simulink model "hinf_arduino"  (R2015a)
settings: Solver=ode3  StartTime=0.0  StopTime=10.0  FixedStep=1/200  RelTol=1e-3
values from neighbouring files (symbols this model uses):
  Hinf = ss(Hinf_red)    [controller_parameters.m]
libraries: PoliArd x9, simulink x6
settings Model: ExtModeTrigDuration=2  Creator=GSavaia  LastModifiedBy=user
settings OptimizationCC: OptimizeModelRefInitCode=on  LifeSpan=1
settings DebuggingCC: UnderspecifiedInitializationDetection=Classic  MergeDetectMultiDrivingBlocksExec=none
settings HardwareCC: ProdLargestAtomicInteger=Long  ProdLargestAtomicFloat=Double  ProdEndianess=LittleEndian  ProdHWDeviceType=ARM Compatible->ARM Cortex
settings RTWCC: SystemTargetFile=realtime.tlc  GenerateMakefile=off  TemplateMakefile=realtime.tmf  Description=Run on Target Hardware  RTWVerbose=off
settings ERTTargetCC: CombineOutputUpdateFcns=off  ExtModeTransport=3  ExtModeMexFile=ext_serial_win32_comm_rtt  ExtModeMexArgs=0 1 9600  ERTSrcFileBannerTemplate=realtime_code_template.cgt  ERTHdrFileBannerTemplate=realtime_code_template.cgt  ERTDataSrcFileTemplate=realtime_code_template.cgt  ERTDataHdrFileTemplate=realtime_code_template.cgt  ERTCustomFileTemplate=realtime_file_process.tlc

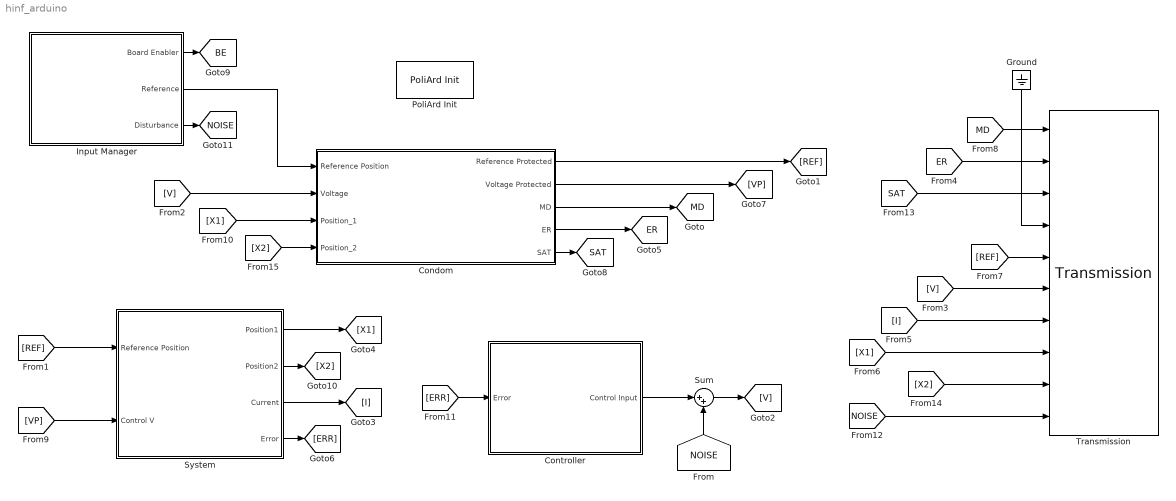
== system hinf_arduino ==
  Condom : Subsystem
  Controller : Subsystem
  Ground : Ground
  Input Manager : Subsystem
  PoliArd Init : PoliArd/PoliArd Init
  Sum : Sum  Inputs=|++
  "System " : Subsystem
  Transmission : PoliArd/Transmission  sample_freq=200  sig_to_send=6
  tag scope: BE=global, ER=global, MD=global, NOISE=global, SAT=global
  wires:
  Condom/1(Reference Protected) -> [REF]
  [REF] -> "System "/1(Reference Position)
  "System "/3(Current) -> [I]
  [V] -> Condom/2(Voltage)
  [V] -> Transmission/6
  [I] -> Transmission/7
  "System "/1(Position1) -> [X1]
  [REF] -> Transmission/5
  [MD] -> Transmission/1
  [VP] -> "System "/2(Control V)
  [X1] -> Condom/3(Position_1)
  [X1] -> Transmission/8
  "System "/4(Error) -> [ERR]
  [ERR] -> Controller/1(Error)
  Condom/2("Voltage Protected ") -> [VP]
  Condom/3(MD) -> [MD]
  Condom/4(ER) -> [ER]
  Ground/1 -> Transmission/4
  [ER] -> Transmission/2
  [SAT] -> Transmission/3
  Condom/5(SAT) -> [SAT]
  Sum/1 -> [V]
  Controller/1(Control Input) -> Sum/1
  [NOISE] -> Sum/2
  Input Manager/1(Board Enabler) -> [BE]
  Input Manager/3(Disturbance) -> [NOISE]
  Input Manager/2(Reference) -> Condom/1(Reference Position)
  "System "/2(Position2) -> [X2]
  [NOISE] -> Transmission/10
  [X2] -> Condom/4(Position_2)
  [X2] -> Transmission/9

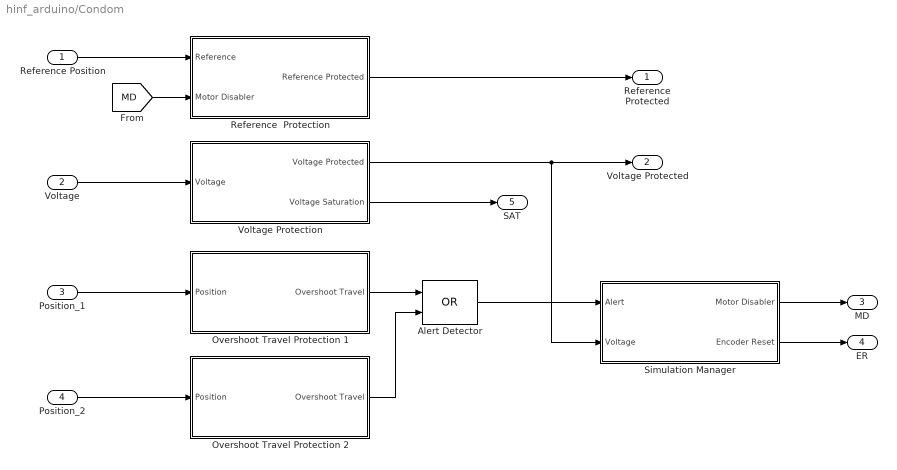
== system hinf_arduino/Condom ==
  Reference Position : Inport
  Voltage : Inport  Port=2
  Position_1 : Inport  Port=3
  Position_2 : Inport  Port=4
  Alert Detector : Logic  Operator=OR  AllPortsSameDT=off  OutDataTypeStr=boolean
  Overshoot Travel Protection 1 : Subsystem
  Overshoot Travel Protection 2 : Subsystem
  Reference  Protection : Subsystem
  Simulation Manager : Subsystem
  Voltage Protection : Subsystem
  Reference Protected : Outport
  "Voltage Protected " : Outport  Port=2
  MD : Outport  Port=3
  ER : Outport  Port=4
  SAT : Outport  Port=5
  wires:
  Reference Position/1 -> Reference  Protection/1("Reference ")
  Position_1/1 -> Overshoot Travel Protection 1/1("Position ")
  Overshoot Travel Protection 1/1(Overshoot Travel) -> Alert Detector/1
  Voltage/1 -> Voltage Protection/1("Voltage ")
  Voltage Protection/1(Voltage Protected) -> Simulation Manager/2(Voltage), "Voltage Protected "/1
  Reference  Protection/1(Reference Protected) -> Reference Protected/1
  Alert Detector/1 -> Simulation Manager/1(Alert)
  Simulation Manager/2(Encoder Reset) -> ER/1
  Simulation Manager/1(Motor Disabler) -> MD/1
  [MD] -> Reference  Protection/2(Motor Disabler)
  Voltage Protection/2(Voltage Saturation) -> SAT/1
  Position_2/1 -> Overshoot Travel Protection 2/1("Position ")
  Overshoot Travel Protection 2/1(Overshoot Travel) -> Alert Detector/2

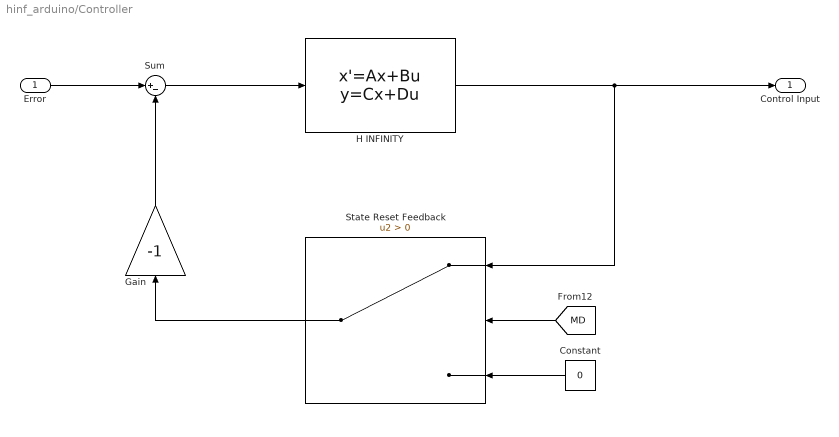
== system hinf_arduino/Controller ==
  Error : Inport
  Constant : Constant  Value=0
  Gain : Gain  Gain=-1
  H INFINITY : StateSpace  A=Hinf.A  B=Hinf.B  C=Hinf.C  D=Hinf.D  X0=0
  State Reset Feedback : Switch  Criteria=u2 > Threshold
  Sum : Sum  Inputs=|+-
  Control Input : Outport
  wires:
  H INFINITY/1 -> State Reset Feedback/1, Control Input/1
  Error/1 -> Sum/1
  Sum/1 -> H INFINITY/1
  Constant/1 -> State Reset Feedback/3
  Gain/1 -> Sum/2
  State Reset Feedback/1 -> Gain/1
  [MD] -> State Reset Feedback/2

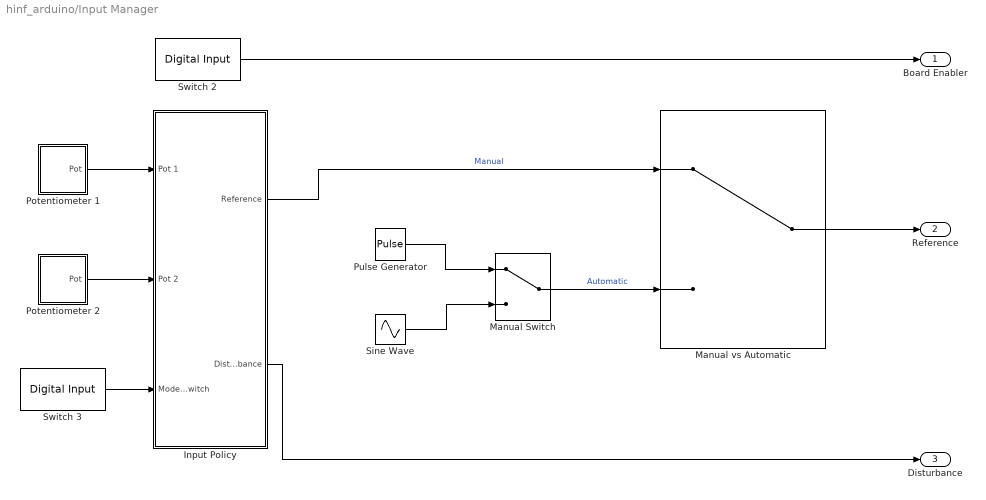
== system hinf_arduino/Input Manager ==
  Input Policy : Subsystem
  Manual vs Automatic : ManualSwitch
  Manual Switch : ManualSwitch
  Potentiometer 1 : Subsystem
  Potentiometer 2 : Subsystem
  Pulse Generator : DiscretePulseGenerator  PulseType=Time based  Amplitude=2  Period=10  PulseWidth=50
  Sine Wave : Sin  Amplitude=0.5  Bias=0.7  Frequency=pi  SampleTime=0
  Switch 2 : PoliArd/Digital Input  DI_pin=2  DIsample=-1
  Switch 3 : PoliArd/Digital Input  DI_pin=3  DIsample=-1
  Board Enabler : Outport
  Reference : Outport  Port=2
  Disturbance : Outport  Port=3
  wires:
  Switch 2/1 -> Board Enabler/1
  Switch 3/1 -> Input Policy/3(Mode Switch)
  Pulse Generator/1 -> Manual Switch/1
  Sine Wave/1 -> Manual Switch/2
  Potentiometer 1/1(Pot) -> Input Policy/1(Pot 1)
  Potentiometer 2/1(Pot) -> Input Policy/2(Pot 2)
  Input Policy/1(Reference) -> Manual vs Automatic/1  "Manual"
  Manual Switch/1 -> Manual vs Automatic/2  "Automatic"
  Input Policy/2(Disturbance) -> Disturbance/1
  Manual vs Automatic/1 -> Reference/1

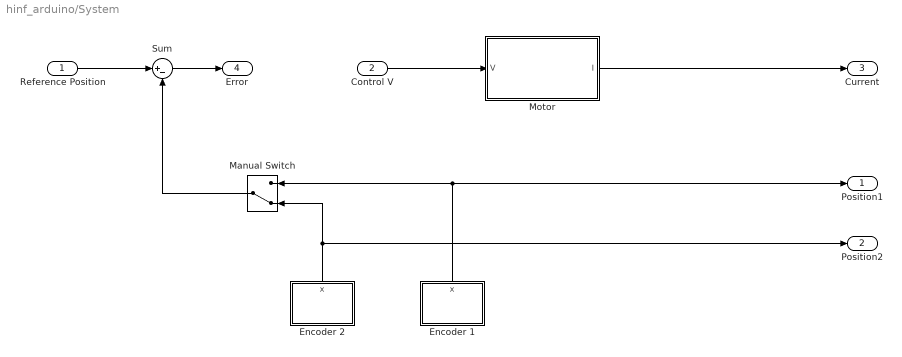
== system hinf_arduino/System  ==
  Reference Position : Inport
  Control V : Inport  Port=2
  "Encoder 1 " : Subsystem
  Encoder 2 : Subsystem
  Manual Switch : ManualSwitch  CurrentSetting=0
  Motor : Subsystem
  Sum : Sum  Inputs=|+-
  Position1 : Outport
  Position2 : Outport  Port=2
  Current : Outport  Port=3
  Error : Outport  Port=4
  wires:
  Reference Position/1 -> Sum/1
  Motor/1(I) -> Current/1
  Sum/1 -> Error/1
  Control V/1 -> Motor/1(V)
  Manual Switch/1 -> Sum/2
  Encoder 2/1(x) -> Position2/1, Manual Switch/2
  "Encoder 1 "/1(x) -> Manual Switch/1, Position1/1

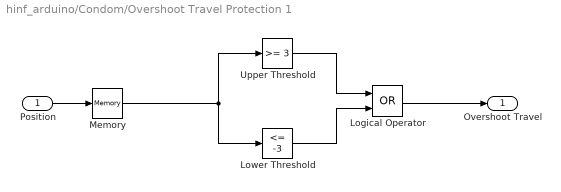
== system hinf_arduino/Condom/Overshoot Travel Protection 1 ==
  "Position " : Inport
  Logical Operator : Logic  Operator=OR  AllPortsSameDT=off  OutDataTypeStr=boolean
  Lower Threshold : simulink/Logic and Bit Operations/Compare To Constant  relop=<=  const=-3  OutDataTypeStr=boolean
  Memory : Memory  InheritSampleTime=on
  Upper Threshold : simulink/Logic and Bit Operations/Compare To Constant  relop=>=  const=3  OutDataTypeStr=boolean
  Overshoot Travel : Outport
  wires:
  Logical Operator/1 -> Overshoot Travel/1
  Lower Threshold/1 -> Logical Operator/2
  Upper Threshold/1 -> Logical Operator/1
  "Position "/1 -> Memory/1
  Memory/1 -> Lower Threshold/1, Upper Threshold/1

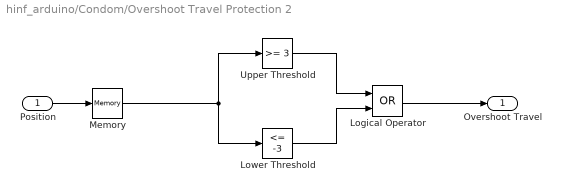
== system hinf_arduino/Condom/Overshoot Travel Protection 2 ==
  "Position " : Inport
  Logical Operator : Logic  Operator=OR  AllPortsSameDT=off  OutDataTypeStr=boolean
  Lower Threshold : simulink/Logic and Bit Operations/Compare To Constant  relop=<=  const=-3  OutDataTypeStr=boolean
  Memory : Memory  InheritSampleTime=on
  Upper Threshold : simulink/Logic and Bit Operations/Compare To Constant  relop=>=  const=3  OutDataTypeStr=boolean
  Overshoot Travel : Outport
  wires:
  Logical Operator/1 -> Overshoot Travel/1
  Lower Threshold/1 -> Logical Operator/2
  Upper Threshold/1 -> Logical Operator/1
  "Position "/1 -> Memory/1
  Memory/1 -> Lower Threshold/1, Upper Threshold/1

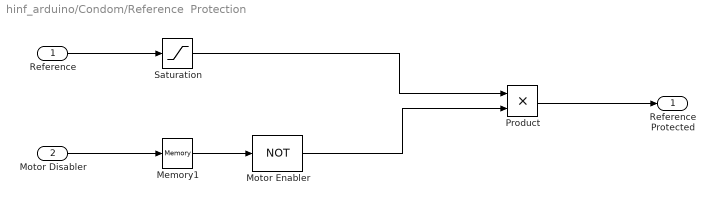
== system hinf_arduino/Condom/Reference  Protection ==
  "Reference " : Inport
  Motor Disabler : Inport  Port=2
  Memory1 : Memory  X0=1  InheritSampleTime=on
  Motor Enabler : Logic  Operator=NOT  Inputs=1  AllPortsSameDT=off  OutDataTypeStr='double'
  Product : Product
  Saturation : Saturate  UpperLimit=3  LowerLimit=-3
  Reference Protected : Outport
  wires:
  "Reference "/1 -> Saturation/1
  Saturation/1 -> Product/1
  Motor Enabler/1 -> Product/2
  Memory1/1 -> Motor Enabler/1
  Product/1 -> Reference Protected/1
  Motor Disabler/1 -> Memory1/1

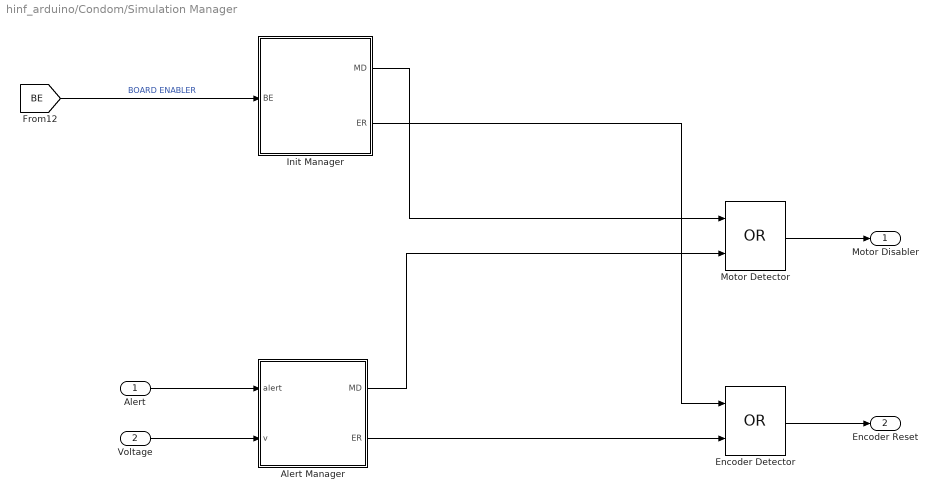
== system hinf_arduino/Condom/Simulation Manager ==
  Alert : Inport
  Voltage : Inport  Port=2
  Alert Manager : Stateflow chart  TreatAsAtomicUnit=on
  Encoder Detector : Logic  Operator=OR  AllPortsSameDT=off  OutDataTypeStr=boolean
  Init Manager : Stateflow chart  TreatAsAtomicUnit=on
  Motor Detector : Logic  Operator=OR  AllPortsSameDT=off  OutDataTypeStr=boolean
  Motor Disabler : Outport
  Encoder Reset : Outport  Port=2
  wires:
  [BE] -> Init Manager/1(BE)  "BOARD ENABLER"
  Motor Detector/1 -> Motor Disabler/1
  Encoder Detector/1 -> Encoder Reset/1
  Init Manager/1(MD) -> Motor Detector/1
  Alert Manager/1(MD) -> Motor Detector/2
  Init Manager/2(ER) -> Encoder Detector/1
  Alert Manager/2(ER) -> Encoder Detector/2
  Alert/1 -> Alert Manager/1(alert)
  Voltage/1 -> Alert Manager/2(v)

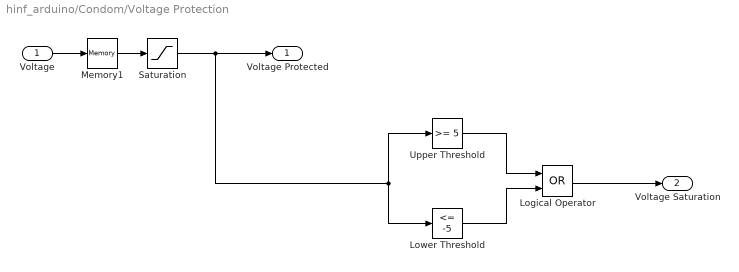
== system hinf_arduino/Condom/Voltage Protection ==
  "Voltage " : Inport
  Logical Operator : Logic  Operator=OR  AllPortsSameDT=off  OutDataTypeStr=boolean
  Lower Threshold : simulink/Logic and Bit Operations/Compare To Constant  relop=<=  const=-5  OutDataTypeStr=boolean
  Memory1 : Memory  InheritSampleTime=on
  Saturation : Saturate  UpperLimit=5  LowerLimit=-5
  Upper Threshold : simulink/Logic and Bit Operations/Compare To Constant  relop=>=  const=5  OutDataTypeStr=boolean
  Voltage Protected : Outport
  Voltage Saturation : Outport  Port=2
  wires:
  "Voltage "/1 -> Memory1/1
  Logical Operator/1 -> Voltage Saturation/1
  Lower Threshold/1 -> Logical Operator/2
  Upper Threshold/1 -> Logical Operator/1
  Saturation/1 -> Lower Threshold/1, Upper Threshold/1, Voltage Protected/1
  Memory1/1 -> Saturation/1

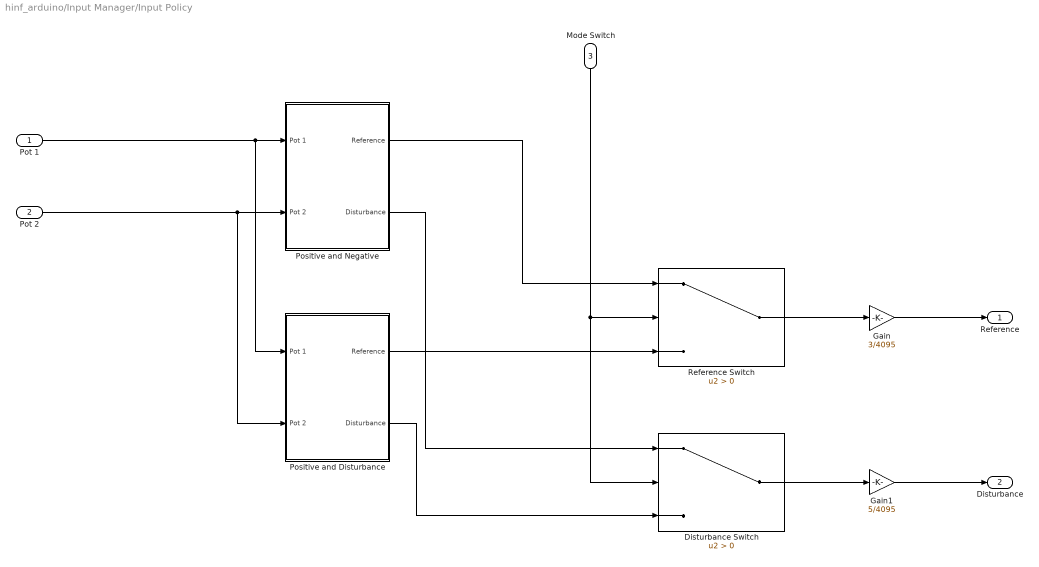
== system hinf_arduino/Input Manager/Input Policy ==
  Pot 1 : Inport
  Pot 2 : Inport  Port=2
  Mode Switch : Inport  Port=3
  Disturbance Switch : Switch  Criteria=u2 > Threshold
  Gain : Gain  Gain=3/4095
  Gain1 : Gain  Gain=5/4095
  Positive and Disturbance : Subsystem
  Positive and Negative : Subsystem
  Reference Switch : Switch  Criteria=u2 > Threshold
  Reference : Outport
  Disturbance : Outport  Port=2
  wires:
  Pot 1/1 -> Positive and Disturbance/1(Pot 1), Positive and Negative/1(Pot 1)
  Pot 2/1 -> Positive and Disturbance/2(Pot 2), Positive and Negative/2(Pot 2)
  Mode Switch/1 -> Reference Switch/2, Disturbance Switch/2
  Reference Switch/1 -> Gain/1
  Disturbance Switch/1 -> Gain1/1
  Positive and Negative/1(Reference) -> Reference Switch/1
  Positive and Disturbance/1(Reference) -> Reference Switch/3
  Positive and Negative/2(Disturbance) -> Disturbance Switch/1
  Positive and Disturbance/2(Disturbance) -> Disturbance Switch/3
  Gain/1 -> Reference/1
  Gain1/1 -> Disturbance/1

== system hinf_arduino/Input Manager/Potentiometer 1 ==
  Analog Input : PoliArd/Analog Input  AIpin_mask=8  AIsample=-1
  Data Type Conversion1 : DataTypeConversion
  Transfer Fcn : TransferFcn  Numerator=1  Denominator=[1/(2*pi*5) 1]
  Pot : Outport
  wires:
  Analog Input/1 -> Data Type Conversion1/1
  Transfer Fcn/1 -> Pot/1
  Data Type Conversion1/1 -> Transfer Fcn/1

== system hinf_arduino/Input Manager/Potentiometer 2 ==
  Analog Input : PoliArd/Analog Input  AIpin_mask=9  AIsample=-1
  Data Type Conversion1 : DataTypeConversion
  Transfer Fcn : TransferFcn  Numerator=1  Denominator=[1/(2*pi*5) 1]
  Pot : Outport
  wires:
  Analog Input/1 -> Data Type Conversion1/1
  Transfer Fcn/1 -> Pot/1
  Data Type Conversion1/1 -> Transfer Fcn/1

== system hinf_arduino/System /Encoder 1  ==
  Encoder : PoliArd/Encoder  EncoderID=1  dt_enc=1/200
  encoder-to-cm : Gain  Gain=1/560
  x : Outport
  wires:
  Encoder/1 -> encoder-to-cm/1
  [ER] -> Encoder/1
  encoder-to-cm/1 -> x/1

== system hinf_arduino/System /Encoder 2 ==
  Encoder : PoliArd/Encoder  EncoderID=4  dt_enc=1/200
  encoder-to-cm : Gain  Gain=1/560
  x : Outport
  wires:
  Encoder/1 -> encoder-to-cm/1
  [ER] -> Encoder/1
  encoder-to-cm/1 -> x/1

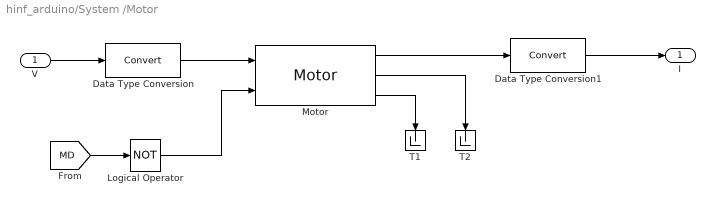
== system hinf_arduino/System /Motor ==
  V : Inport
  Data Type Conversion : DataTypeConversion
  Data Type Conversion1 : DataTypeConversion
  Logical Operator : Logic  Operator=NOT  AllPortsSameDT=off  OutDataTypeStr=boolean
  Motor : PoliArd/Motor  MotorID=2  DC_bus_mask=12  dt_mot=1/200
  T1 : Terminator
  T2 : Terminator
  I : Outport
  wires:
  Data Type Conversion/1 -> Motor/1
  V/1 -> Data Type Conversion/1
  Motor/3 -> T1/1
  Motor/2 -> T2/1
  Motor/1 -> Data Type Conversion1/1
  Data Type Conversion1/1 -> I/1
  Logical Operator/1 -> Motor/2
  [MD] -> Logical Operator/1

== system hinf_arduino/Input Manager/Input Policy/Positive and Disturbance ==
  Pot 1 : Inport
  Pot 2 : Inport  Port=2
  Reference : Outport
  Disturbance : Outport  Port=2
  wires:
  Pot 1/1 -> Reference/1
  Pot 2/1 -> Disturbance/1

== system hinf_arduino/Input Manager/Input Policy/Positive and Negative ==
  Pot 1 : Inport
  Pot 2 : Inport  Port=2
  Add : Sum  Inputs=+-
  Constant : Constant  Value=0
  Reference : Outport
  Disturbance : Outport  Port=2
  wires:
  Add/1 -> Reference/1
  Constant/1 -> Disturbance/1
  Pot 2/1 -> Add/2
  Pot 1/1 -> Add/1

== stateflow chart hinf_arduino/Condom/Simulation Manager/Init Manager ==
  state STOP
    entry:
    MD = 1;
    ER = 1;
  state OPERATIVE
    entry:
    MD = 0;
    ER = 0;
  state INIT
    entry:
    MD = 1;
    ER  = 1;
  (default) -> STOP
  OPERATIVE -> STOP : [BE==0]
  STOP -> INIT : [BE==1]
  INIT -> OPERATIVE : after(3, sec)
  data: MD output; ER output; BE input

== stateflow chart hinf_arduino/Condom/Simulation Manager/Alert Manager ==
  state OK
    entry:
    MD=0;
    ER=0;
  state ALERT
    entry:
    MD=1;
    ER=1;
  (default) -> OK
  OK -> ALERT : [alert==1]
  ALERT -> OK : [abs(v)<0.3]
  data: alert input; v input; MD output; ER output
